simulink model "vegas13_fastnettest_250mhz_r1"  (Simulink 7.4)
settings: Solver=ode45  StartTime=0.0  StopTime=20000  RelTol=1e-3
undefined symbols (not defined in the file or in its folder): ROACH
libraries: xbsIndex_r4 x179, xps_library x20, casper_library_misc x18, dspsigops x16, casper_library_flow_control x4
(part 1 of 3)
settings Model: Creator=dave  LastModifiedBy=sscott
settings OptimizationCC: InitFltsAndDblsToZero=on

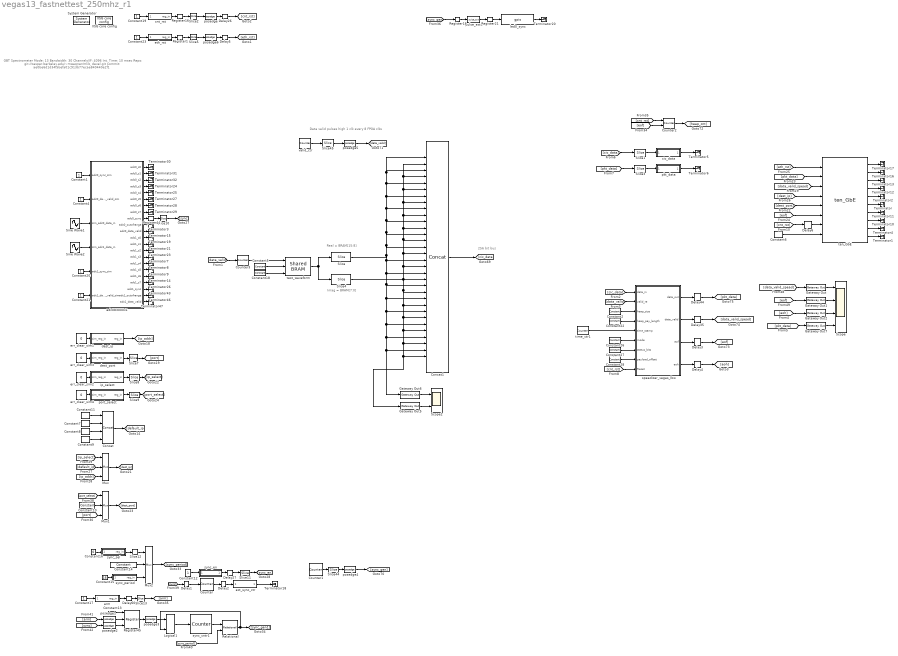
== system vegas13_fastnettest_250mhz_r1 ==
  note: GBT Spectrometer
      | Mode: 13
      | Bandwidth: 30
      | Channels/IF: 4096
      | Int. Time: 10 msec
      | Repo: git://casper.berkeley.edu/~mwagner/mlib_devel.git
      | Commit: ae0be6d1d34f5befa01c913b77ecae840440e2f1
  note: Data valid pulses high 1 clk every 8 FPGA clks
  note: 256 bit bus
  note: Real = BRAM[15:8]
  note: Imag = BRAM[7:0]
  " System Generator" : xbsIndex_r4/ System Generator  Tag=genX  SystemSampleTime=-1  xilinxfamily=virtex5  part=xc5vsx95t  speed=-1  package=ff1136  synthesis_tool=XST  clock_wrapper=Clock Enables  directory=./vegas13_fastnettest_250mhz_r1/sysgen  testbench=off  simulink_period=1  sysclk_period=4  dcm_input_clock_period=100  incr_netlist=off  trim_vbits=Everywhere in SubSystem  dbl_ovrd=According to Block Masks  core_generation=According to Block Masks  run_coregen=off  deprecated_control=off  eval_field=0  block_type=sysgen
      settings: block_version=10.1.3
  Concat : xbsIndex_r4/Concat  num_inputs=4  dbl_ovrd=off  block_type=concat
  Concat1 : xbsIndex_r4/Concat  num_inputs=32  dbl_ovrd=off  block_type=concat
  Constant{1,4,20..21} (4 alike) : Constant  OutDataType=sfix(16)  OutScaling=2^0  SampleTime=1
  Constant10 : xbsIndex_r4/Constant  arith_type=Unsigned  const=10145  n_bits=32  bin_pt=0  explicit_period=on  period=1  equ=P=C  opselect=C  inp2=PCIN>>17  opr=+  inp1=P  carry=CIN  dbl_ovrd=off  block_type=constant
  Constant11 : xbsIndex_r4/Constant  arith_type=Unsigned  const=10  n_bits=8  bin_pt=0  explicit_period=on  period=1  equ=P=C  opselect=C  inp2=PCIN>>17  opr=+  inp1=P  carry=CIN  dbl_ovrd=off  block_type=constant
  Constant12 : Constant  OutDataType=fixdt(1, 16)  OutScaling=2^0
  Constant13 : xbsIndex_r4/Constant  arith_type=Boolean  const=1  n_bits=16  bin_pt=14  explicit_period=on  period=1  equ=P=C  opselect=C  inp2=PCIN>>17  opr=+  inp1=P  carry=CIN  dbl_ovrd=off  block_type=constant
  Constant14 : xbsIndex_r4/Constant  arith_type=Unsigned  const=100663295  n_bits=32  bin_pt=0  explicit_period=on  period=1  equ=P=C  opselect=C  inp2=PCIN>>17  opr=+  inp1=P  carry=CIN  dbl_ovrd=off  block_type=constant
  Constant15 : Constant  Value=16  OutDataType=sfix(16)  OutScaling=2^0
  Constant16 : Constant  Value=0  OutDataType=sfix(16)  OutScaling=2^0
  Constant17 : Constant  OutDataType=sfix(16)  OutScaling=2^0
  Constant{5,18,27..28} (4 alike) : xbsIndex_r4/Constant  arith_type=Unsigned  const=0  n_bits=40  bin_pt=0  explicit_period=on  period=1  equ=P=C  opselect=C  inp2=PCIN>>17  opr=+  inp1=P  carry=CIN  dbl_ovrd=off  block_type=constant
  Constant19 : Constant  OutDataType=sfix(16)  OutScaling=2^0
  Constant2 : xbsIndex_r4/Constant  arith_type=Unsigned  const=8192+4*8  n_bits=40  bin_pt=0  explicit_period=on  period=1  equ=P=C  opselect=C  inp2=PCIN>>17  opr=+  inp1=P  carry=CIN  dbl_ovrd=off  block_type=constant
  Constant22 : xbsIndex_r4/Constant  arith_type=Unsigned  const=8192  n_bits=40  bin_pt=0  explicit_period=on  period=1  equ=P=C  opselect=C  inp2=PCIN>>17  opr=+  inp1=P  carry=CIN  dbl_ovrd=off  block_type=constant
  Constant23 : Constant  OutDataType=sfix(16)  OutScaling=2^0
  Constant26 : xbsIndex_r4/Constant  arith_type=Unsigned  const=13  n_bits=40  bin_pt=0  explicit_period=on  period=1  equ=P=C  opselect=C  inp2=PCIN>>17  opr=+  inp1=P  carry=CIN  dbl_ovrd=off  block_type=constant
  Constant6 : xbsIndex_r4/Constant  arith_type=Boolean  const=0  n_bits=1  bin_pt=0  explicit_period=on  period=1  equ=P=C  opselect=C  inp2=PCIN>>17  opr=+  inp1=P  carry=CIN  dbl_ovrd=off  block_type=constant
  Constant7 : xbsIndex_r4/Constant  arith_type=Unsigned  const=0  n_bits=8  bin_pt=0  explicit_period=on  period=1  equ=P=C  opselect=C  inp2=PCIN>>17  opr=+  inp1=P  carry=CIN  dbl_ovrd=off  block_type=constant
  Constant8 : xbsIndex_r4/Constant  arith_type=Unsigned  const=0  n_bits=8  bin_pt=0  explicit_period=on  period=1  equ=P=C  opselect=C  inp2=PCIN>>17  opr=+  inp1=P  carry=CIN  dbl_ovrd=off  block_type=constant
  Constant9 : xbsIndex_r4/Constant  arith_type=Unsigned  const=145  n_bits=8  bin_pt=0  explicit_period=on  period=1  equ=P=C  opselect=C  inp2=PCIN>>17  opr=+  inp1=P  carry=CIN  dbl_ovrd=off  block_type=constant
  Counter : xbsIndex_r4/Counter  cnt_type=Free Running  cnt_to=Inf  operation=Up  start_count=0  cnt_by_val=1  arith_type=Unsigned  n_bits=8  bin_pt=0  load_pin=off  rst=off  en=on  explicit_period=on  period=1  dbl_ovrd=off  use_behavioral_HDL=off  implementation=Fabric  block_type=counter
      settings: block_version=11.4
  Counter1 : xbsIndex_r4/Counter  cnt_type=Free Running  cnt_to=Inf  operation=Up  start_count=0  cnt_by_val=1  arith_type=Unsigned  n_bits=5  bin_pt=0  load_pin=off  rst=off  en=off  explicit_period=on  period=1  dbl_ovrd=off  use_behavioral_HDL=off  implementation=Fabric  block_type=counter
      settings: block_version=11.4
  Counter2 : xbsIndex_r4/Counter  cnt_type=Free Running  cnt_to=Inf  operation=Up  start_count=0  cnt_by_val=1  arith_type=Unsigned  n_bits=40  bin_pt=0  load_pin=off  rst=on  en=on  explicit_period=on  period=1  dbl_ovrd=off  use_behavioral_HDL=off  implementation=Fabric  block_type=counter
      settings: block_version=11.4
  Counter3 : xbsIndex_r4/Counter  cnt_type=Free Running  cnt_to=Inf  operation=Up  start_count=0  cnt_by_val=1  arith_type=Unsigned  n_bits=4  bin_pt=0  load_pin=off  rst=off  en=on  explicit_period=on  period=1  dbl_ovrd=off  use_behavioral_HDL=off  implementation=Fabric  block_type=counter
      settings: block_version=11.4
  Delay1 : xbsIndex_r4/Delay  en=off  latency=8  dbl_ovrd=off  reg_retiming=off  block_type=delay
      settings: block_version=11.4
  Delay2 : xbsIndex_r4/Delay  en=off  latency=8  dbl_ovrd=off  reg_retiming=off  block_type=delay
      settings: block_version=11.4
  Delay26 : xbsIndex_r4/Delay  en=off  latency=8  dbl_ovrd=off  reg_retiming=on  block_type=delay
  Delay27 : xbsIndex_r4/Delay  en=off  latency=8  dbl_ovrd=off  reg_retiming=off  block_type=delay
      settings: block_version=11.4
  Delay{3..4,6,35,44} (5 alike) : xbsIndex_r4/Delay  en=off  latency=1  dbl_ovrd=off  reg_retiming=on  block_type=delay
  Delay5 : xbsIndex_r4/Delay  en=off  latency=8  dbl_ovrd=off  reg_retiming=on  block_type=delay
  Delay60 : xbsIndex_r4/Delay  en=off  latency=2  dbl_ovrd=off  reg_retiming=on  block_type=delay
  Gateway Out{,1..2,5..7} (6 alike) : xbsIndex_r4/Gateway Out  hdl_port=on  timing_constraint=None  locs_specified=off  LOCs={}  block_type=gatewayout
      settings: infoedit="Gateway out block.  Converts Xilinx fixed point inputs into ouputs of type Simulink integer, double, or fixed point.<br><br>Hardware notes:  In hardware these blocks become top level output ports or are discarded, depending on how they are configured."  block_version=11.4
  Logical1 : xbsIndex_r4/Logical  logical_function=OR  inputs=2  en=off  latency=0  precision=Full  arith_type=Unsigned  n_bits=16  bin_pt=0  align_bp=on  dbl_ovrd=off  block_type=logical
  Mux : xbsIndex_r4/Mux  inputs=2  en=off  latency=0  precision=Full  arith_type=Unsigned  n_bits=16  bin_pt=14  quantization=Truncate  overflow=Wrap  dbl_ovrd=off  block_type=mux
      settings: block_version=11.4
  Mux1 : xbsIndex_r4/Mux  inputs=2  en=off  latency=0  precision=Full  arith_type=Unsigned  n_bits=16  bin_pt=14  quantization=Truncate  overflow=Wrap  dbl_ovrd=off  block_type=mux
      settings: block_version=11.4
  Mux2 : xbsIndex_r4/Mux  inputs=2  en=off  latency=0  precision=Full  arith_type=Unsigned  n_bits=16  bin_pt=14  quantization=Truncate  overflow=Wrap  dbl_ovrd=off  block_type=mux
      settings: block_version=11.4
  Register{1,16,18,21,44} (5 alike) : xbsIndex_r4/Register  init=0  rst=off  en=off  dbl_ovrd=off  block_type=register
      settings: block_version=11.4
  Register45 : xbsIndex_r4/Register  init=0  rst=on  en=on  dbl_ovrd=off  block_type=register
      settings: block_version=11.4
  Relational : xbsIndex_r4/Relational  mode=a>=b  en=off  latency=0  dbl_ovrd=off  block_type=relational
      settings: xl_area=[0, 0, 0, 0, 0, 0, 0]  block_version=9.1.01
  Scope : Scope  NumInputPorts=4
      settings: TimeRange=6000  YMin=0~-1~0~0  YMax=1~1~300000000000000~1e+19  MaxDataPoints=1000000
  Scope2 : Scope  NumInputPorts=2
      settings: YMin=0~-5  YMax=1~5  SaveName=ScopeData3  MaxDataPoints=1000000
  Sine Wave1 : Sin  Amplitude=.9  Bias=0  Frequency=2.*pi/4.  Phase=2*pi*240/200  Samples=10  SampleTime=.0625  Offset=0
  Sine Wave2 : Sin  Amplitude=.9  Bias=0  Frequency=2.*pi/4.  Phase=2*pi*240/200  Samples=10  SampleTime=.0625  Offset=0
  Slice : xbsIndex_r4/Slice  nbits=8  boolean_output=off  mode=Lower Bit Location + Width  bit1=0  base1=MSB of Input  bit0=8  base0=LSB of Input  dbl_ovrd=off  block_type=slice
  Slice1 : xbsIndex_r4/Slice  nbits=32  boolean_output=off  mode=Lower Bit Location + Width  bit1=0  base1=MSB of Input  bit0=0  base0=LSB of Input  dbl_ovrd=off  block_type=slice
  Slice{2,5,8..13} (8 alike) : xbsIndex_r4/Slice  nbits=1  boolean_output=on  mode=Lower Bit Location + Width  bit1=0  base1=MSB of Input  bit0=0  base0=LSB of Input  dbl_ovrd=off  block_type=slice
      Slice10 settings: infoedit="Extracts a given range of bits from each input sample and presents it at the output.  The output type is ordinarily unsigned with binary point at zero, but can be Boolean when the slice is one bit wide.<P><P>Hardware notes: In hardware this block costs nothing."  block_version=10.1.3
      Slice12 settings: block_version=10.1.3
      Slice13 settings: infoedit="Extracts a given range of bits from each input sample and presents it at the output.  The output type is ordinarily unsigned with binary point at zero, but can be Boolean when the slice is one bit wide.<P><P>Hardware notes: In hardware this block costs nothing."  block_version=10.1.3
      Slice2 settings: block_version=10.1.3
      Slice5 settings: block_version=10.1.3
      Slice8 settings: block_version=10.1.3
      Slice9 settings: block_version=10.1.3
  Slice3 : xbsIndex_r4/Slice  nbits=32  boolean_output=off  mode=Lower Bit Location + Width  bit1=0  base1=MSB of Input  bit0=0  base0=LSB of Input  dbl_ovrd=off  block_type=slice
  Slice4 : xbsIndex_r4/Slice  nbits=8  boolean_output=off  mode=Lower Bit Location + Width  bit1=0  base1=LSB of Input  bit0=0  base0=LSB of Input  dbl_ovrd=off  block_type=slice
  Slice44 : xbsIndex_r4/Slice  nbits=1  boolean_output=on  mode=Upper Bit Location + Width  bit1=0  base1=MSB of Input  bit0=0  base0=LSB of Input  dbl_ovrd=off  block_type=slice
  Slice45 : xbsIndex_r4/Slice  nbits=1  boolean_output=on  mode=Upper Bit Location + Width  bit1=0  base1=MSB of Input  bit0=0  base0=LSB of Input  dbl_ovrd=off  block_type=slice
  Slice7 : xbsIndex_r4/Slice  nbits=16  boolean_output=off  mode=Lower Bit Location + Width  bit1=0  base1=MSB of Input  bit0=0  base0=LSB of Input  dbl_ovrd=off  block_type=slice
      settings: infoedit="Extracts a given range of bits from each input sample and presents it at the output.  The output type is ordinarily unsigned with binary point at zero, but can be Boolean when the slice is one bit wide.<P><P>Hardware notes: In hardware this block costs nothing."  block_version=10.1.3
  Terminator{,1..21,23..32,43,46..47} (35 alike) : Terminator
  XSG core config : xps_library/XSG core config  Tag=xps:xsg  SystemSampleTime=-1  hw_sys=ROACH:sx95t  ibob_linux=off  clk_src=adc0_clk  iBOB_clk_src=adc0_clk  BEE2_ctrl_clk_src=sys_clk  BEE2_usr_clk_src=sys_clk  ROACH_clk_src=adc0_clk  CORR_clk_src=sys_clk  gpio_clk_io_group=iBOB:sma  gpio_clk_bit_index=0  clk_rate=250  sample_period=1  synthesis_tool=XST  mpc_type=powerpc440_ext
  adc083000x1 : Subsystem  Tag=xps:adc083000x2  AncestorBlock=xps_library/adc083000x2  mask(adc_083000x2){use_adc0=on, use_adc1=on, demux_adc=off, clock_sync=off, verbose=off, using_ctrl=on, adc_clk_rate=1000, sample_period=1, bit_width=8}
      mask prompts: use_adc0 "Use ZD0K0?"; use_adc1 "Use ZDOK1?"; demux_adc "Demux ADCs by 2?"; clock_sync "Interleave 2 ADC boards?"; verbose "Verbose Block Creation?"; using_ctrl "Add ports for control registers?"; adc_clk_rate "ADC clock rate (MHz)"; sample_period "Sample Period"; bit_width "Output Bit Width"
      mask help:
      | The ADC block converts analog inputs to digital outputs.
      | Every clock cycle, the inputs are sampled and digitized to
      | 8 bit binary point numbers in the range of [-1, 1).
      |
      | Online block-specific documentation: http://casper.berkeley.edu/wiki/Adc083000
      mask init:
      | adc083000_mask;
      mask Help: eval('xlWeb([getenv(''MLIB_ROOT''), ''\doc\html\sys_adc\sys_adc.html''])')
  arm : Subsystem  Tag=xps:sw_reg  mask{io_dir=From Processor, arith_type=Unsigned, bitwidth=32, bin_pt=0, sample_period=1, latency=0}
      link override convert: arith_type=Unsigned  n_bits=32  bin_pt=0
      link override r_spec_2048_r102_cnt_rst_user_data_out: arith_type=Unsigned  n_bits=32  bin_pt=0  period=1
      link override r_spec_2048_r102_nosim_cnt_rst_user_data_out: arith_type=Unsigned  n_bits=32  bin_pt=0  period=1
      link override r_spec_2048_r103_cnt_rst_user_data_out: arith_type=Unsigned  n_bits=32  bin_pt=0  period=1
      link override roach_spec_no10gbe_sync_cnt_rst_user_data_out: arith_type=Unsigned  n_bits=32  bin_pt=0  period=1
      link override roach_spec_rst_cnt_user_data_out: arith_type=Unsigned  n_bits=32  bin_pt=0  period=1
      link override roach_spec_rst_sync_cnt_user_data_out: arith_type=Unsigned  n_bits=32  bin_pt=0  period=1
      mask prompts: io_dir "I/O direction"; arith_type "Data Type"; bitwidth "Data bitwidth"; bin_pt "Data binary point"; sample_period "Sample period"
      mask init:
      | gw_name = clear_name(gcb);
      | config.source = str2func('software_register_init');
      | config.toplevel = gcb;
      | xBlock( config, {io_dir, arith_type, bitwidth, bin_pt, ... 
      |     sample_period, gw_name, latency});
      mask StyleString: popup(From Processor|To Processor),popup(Unsigned|Signed  (2's comp)),edit,edit,edit,edit
  cic_data : Subsystem  Tag=xps:sw_reg  mask{io_dir=To Processor, arith_type=Unsigned, bitwidth=32, bin_pt=0, sample_period=1, latency=0}
      mask prompts: io_dir "I/O direction"; arith_type "Data Type"; bitwidth "Data bitwidth"; bin_pt "Data binary point"; sample_period "Sample period"
      mask init:
      | gw_name = clear_name(gcb);
      | config.source = str2func('software_register_init');
      | config.toplevel = gcb;
      | xBlock( config, {io_dir, arith_type, bitwidth, bin_pt, ... 
      |     sample_period, gw_name, latency});
      mask StyleString: popup(From Processor|To Processor),popup(Unsigned|Signed  (2's comp)),edit,edit,edit,edit
  cnt_rst : Subsystem  Tag=xps:sw_reg  mask{io_dir=From Processor, arith_type=Unsigned, bitwidth=32, bin_pt=0, sample_period=1, latency=0}
      link override convert: arith_type=Unsigned  n_bits=32  bin_pt=0
      link override r_spec_2048_r102_cnt_rst_user_data_out: arith_type=Unsigned  n_bits=32  bin_pt=0  period=1
      link override r_spec_2048_r102_nosim_cnt_rst_user_data_out: arith_type=Unsigned  n_bits=32  bin_pt=0  period=1
      link override r_spec_2048_r103_cnt_rst_user_data_out: arith_type=Unsigned  n_bits=32  bin_pt=0  period=1
      link override roach_spec_no10gbe_sync_cnt_rst_user_data_out: arith_type=Unsigned  n_bits=32  bin_pt=0  period=1
      link override roach_spec_rst_cnt_user_data_out: arith_type=Unsigned  n_bits=32  bin_pt=0  period=1
      link override roach_spec_rst_sync_cnt_user_data_out: arith_type=Unsigned  n_bits=32  bin_pt=0  period=1
      mask prompts: io_dir "I/O direction"; arith_type "Data Type"; bitwidth "Data bitwidth"; bin_pt "Data binary point"; sample_period "Sample period"
      mask init:
      | gw_name = clear_name(gcb);
      | config.source = str2func('software_register_init');
      | config.toplevel = gcb;
      | xBlock( config, {io_dir, arith_type, bitwidth, bin_pt, ... 
      |     sample_period, gw_name, latency});
      mask StyleString: popup(From Processor|To Processor),popup(Unsigned|Signed  (2's comp)),edit,edit,edit,edit
  dest_ip : Subsystem  Tag=xps:sw_reg  mask{io_dir=From Processor, arith_type=Unsigned, bitwidth=32, bin_pt=0, sample_period=1, latency=0}
      link override r_10gbe_demo_dest_ip_user_data_out: arith_type=Unsigned  n_bits=32  bin_pt=0  period=1
      link override r_10gbe_test_dest_ip_user_data_out: arith_type=Unsigned  n_bits=32  bin_pt=0  period=1
      link override r_xaui_test_cnt_rst_user_data_out: arith_type=Unsigned  n_bits=32  bin_pt=0  period=1
      mask prompts: io_dir "I/O direction"; arith_type "Data Type"; bitwidth "Data bitwidth"; bin_pt "Data binary point"; sample_period "Sample period"
      mask init:
      | gw_name = clear_name(gcb);
      | config.source = str2func('software_register_init');
      | config.toplevel = gcb;
      | xBlock( config, {io_dir, arith_type, bitwidth, bin_pt, ... 
      |     sample_period, gw_name, latency});
      mask StyleString: popup(From Processor|To Processor),popup(Unsigned|Signed  (2's comp)),edit,edit,edit,edit
  dest_port : Subsystem  Tag=xps:sw_reg  mask{io_dir=From Processor, arith_type=Unsigned, bitwidth=32, bin_pt=0, sample_period=1, latency=0}
      link override r_10gbe_demo_dest_port_user_data_out: arith_type=Unsigned  n_bits=32  bin_pt=0  period=1
      link override r_10gbe_test_dest_port_user_data_out: arith_type=Unsigned  n_bits=32  bin_pt=0  period=1
      link override r_xaui_test_cnt_rst_user_data_out: arith_type=Unsigned  n_bits=32  bin_pt=0  period=1
      mask prompts: io_dir "I/O direction"; arith_type "Data Type"; bitwidth "Data bitwidth"; bin_pt "Data binary point"; sample_period "Sample period"
      mask init:
      | gw_name = clear_name(gcb);
      | config.source = str2func('software_register_init');
      | config.toplevel = gcb;
      | xBlock( config, {io_dir, arith_type, bitwidth, bin_pt, ... 
      |     sample_period, gw_name, latency});
      mask StyleString: popup(From Processor|To Processor),popup(Unsigned|Signed  (2's comp)),edit,edit,edit,edit
  err_clear_sim{1..4} (4 alike) : Constant  Value=0  OutDataType=sfix(16)  OutScaling=2^0
  eth_rst : Subsystem  Tag=xps:sw_reg  mask{io_dir=From Processor, arith_type=Unsigned, bitwidth=32, bin_pt=0, sample_period=1, latency=0}
      link override convert: arith_type=Unsigned  n_bits=32  bin_pt=0
      link override r_spec_2048_r102_cnt_rst_user_data_out: arith_type=Unsigned  n_bits=32  bin_pt=0  period=1
      link override r_spec_2048_r102_nosim_cnt_rst_user_data_out: arith_type=Unsigned  n_bits=32  bin_pt=0  period=1
      link override r_spec_2048_r103_cnt_rst_user_data_out: arith_type=Unsigned  n_bits=32  bin_pt=0  period=1
      link override roach_spec_no10gbe_sync_cnt_rst_user_data_out: arith_type=Unsigned  n_bits=32  bin_pt=0  period=1
      link override roach_spec_rst_cnt_user_data_out: arith_type=Unsigned  n_bits=32  bin_pt=0  period=1
      link override roach_spec_rst_sync_cnt_user_data_out: arith_type=Unsigned  n_bits=32  bin_pt=0  period=1
      mask prompts: io_dir "I/O direction"; arith_type "Data Type"; bitwidth "Data bitwidth"; bin_pt "Data binary point"; sample_period "Sample period"
      mask init:
      | gw_name = clear_name(gcb);
      | config.source = str2func('software_register_init');
      | config.toplevel = gcb;
      | xBlock( config, {io_dir, arith_type, bitwidth, bin_pt, ... 
      |     sample_period, gw_name, latency});
      mask StyleString: popup(From Processor|To Processor),popup(Unsigned|Signed  (2's comp)),edit,edit,edit,edit
  ext_sync_ctr : Subsystem  Tag=xps:sw_reg  mask{io_dir=To Processor, arith_type=Unsigned, bitwidth=32, bin_pt=0, sample_period=1, latency=0}
      mask prompts: io_dir "I/O direction"; arith_type "Data Type"; bitwidth "Data bitwidth"; bin_pt "Data binary point"; sample_period "Sample period"
      mask init:
      | gw_name = clear_name(gcb);
      | config.source = str2func('software_register_init');
      | config.toplevel = gcb;
      | xBlock( config, {io_dir, arith_type, bitwidth, bin_pt, ... 
      |     sample_period, gw_name, latency});
      mask StyleString: popup(From Processor|To Processor),popup(Unsigned|Signed  (2's comp)),edit,edit,edit,edit
  ip_select : Subsystem  Tag=xps:sw_reg  mask{io_dir=From Processor, arith_type=Unsigned, bitwidth=32, bin_pt=0, sample_period=1, latency=0}
      link override r_10gbe_demo_gbe_core_rst_user_data_out: arith_type=Unsigned  n_bits=32  bin_pt=0  period=1
      link override r_10gbe_test_cnt_rst_user_data_out: arith_type=Unsigned  n_bits=32  bin_pt=0  period=1
      link override r_10gbe_test_gbe_core_rst_user_data_out: arith_type=Unsigned  n_bits=32  bin_pt=0  period=1
      link override r_xaui_test_cnt_rst_user_data_out: arith_type=Unsigned  n_bits=32  bin_pt=0  period=1
      mask prompts: io_dir "I/O direction"; arith_type "Data Type"; bitwidth "Data bitwidth"; bin_pt "Data binary point"; sample_period "Sample period"
      mask init:
      | gw_name = clear_name(gcb);
      | config.source = str2func('software_register_init');
      | config.toplevel = gcb;
      | xBlock( config, {io_dir, arith_type, bitwidth, bin_pt, ... 
      |     sample_period, gw_name, latency});
      mask StyleString: popup(From Processor|To Processor),popup(Unsigned|Signed  (2's comp)),edit,edit,edit,edit
  led0_sync : xps_library/gpio  Tag=xps:gpio  SystemSampleTime=-1  io_group=ROACH:led  io_dir=out  arith_type=Boolean  bitwidth=1  bin_pt=0  bit_index=0  sample_period=1  use_single_ended=off  use_ddr=off  reg_iob=on  reg_clk_phase=0  termination=None
      link override convert: arith_type=Boolean  n_bits=1  bin_pt=0
  pkt_data : Subsystem  Tag=xps:sw_reg  mask{io_dir=To Processor, arith_type=Unsigned, bitwidth=32, bin_pt=0, sample_period=1, latency=0}
      mask prompts: io_dir "I/O direction"; arith_type "Data Type"; bitwidth "Data bitwidth"; bin_pt "Data binary point"; sample_period "Sample period"
      mask init:
      | gw_name = clear_name(gcb);
      | config.source = str2func('software_register_init');
      | config.toplevel = gcb;
      | xBlock( config, {io_dir, arith_type, bitwidth, bin_pt, ... 
      |     sample_period, gw_name, latency});
      mask StyleString: popup(From Processor|To Processor),popup(Unsigned|Signed  (2's comp)),edit,edit,edit,edit
  port_select : Subsystem  Tag=xps:sw_reg  mask{io_dir=From Processor, arith_type=Unsigned, bitwidth=32, bin_pt=0, sample_period=1, latency=0}
      link override r_10gbe_demo_gbe_core_rst_user_data_out: arith_type=Unsigned  n_bits=32  bin_pt=0  period=1
      link override r_10gbe_test_cnt_rst_user_data_out: arith_type=Unsigned  n_bits=32  bin_pt=0  period=1
      link override r_10gbe_test_gbe_core_rst_user_data_out: arith_type=Unsigned  n_bits=32  bin_pt=0  period=1
      link override r_xaui_test_cnt_rst_user_data_out: arith_type=Unsigned  n_bits=32  bin_pt=0  period=1
      mask prompts: io_dir "I/O direction"; arith_type "Data Type"; bitwidth "Data bitwidth"; bin_pt "Data binary point"; sample_period "Sample period"
      mask init:
      | gw_name = clear_name(gcb);
      | config.source = str2func('software_register_init');
      | config.toplevel = gcb;
      | xBlock( config, {io_dir, arith_type, bitwidth, bin_pt, ... 
      |     sample_period, gw_name, latency});
      mask StyleString: popup(From Processor|To Processor),popup(Unsigned|Signed  (2's comp)),edit,edit,edit,edit
  posedge{,1..6} (7 alike) : casper_library_misc/posedge  Tag=Rising Edge Detector  SystemSampleTime=-1
  pulse_ext1 : casper_library_misc/pulse_ext  SystemSampleTime=-1  pulse_len=2^24
  speadizer_vegas_lbw : Subsystem  AncestorBlock=gbt_library/speadizer_vegas_lbw  mask(speadizer_vegas){spead_msw=24, spead_lsw=40, num_items=4, num_payloads=1, pktzr_waste_time=3, data_input_width=256}
      mask prompts: spead_msw "Num bits for SPEAD Item ID"; spead_lsw "Num bits for SPEAD Item value"; num_items "Number of items (+5)"; num_payloads "Number of packets per heap"; pktzr_waste_time "Packetizer waste time"; data_input_width "Data input width"
      mask help:
      | The size of the heap and payload are in Bytes.
      | If there is one packet per heap then payload_offset is 0.
      | All the input must be not longer than 40 bits.
      mask init:
      | speadizer_vegas_init(gcb, 'spead_msw', spead_msw, 'spead_lsw', spead_lsw, 'num_items', num_items, 'num_payloads', num_payloads, 'pktzr_waste_time', pktzr_waste_time, 'data_input_width', data_input_width)
  sync_cntr1 : xbsIndex_r4/Counter  cnt_type=Free Running  cnt_to=1023  operation=Up  start_count=0  cnt_by_val=1  arith_type=Unsigned  n_bits=10  bin_pt=0  load_pin=off  rst=on  en=off  explicit_period=on  period=1  dbl_ovrd=off  use_behavioral_HDL=off  implementation=Fabric  use_rpm=on  block_type=counter
      settings: xl_area=[0, 0, 0, 0, 0, 0, 0]  block_version=9.1.01
  sync_en : Subsystem  Tag=xps:sw_reg  mask{io_dir=From Processor, arith_type=Unsigned, bitwidth=32, bin_pt=0, sample_period=1, latency=0}
      mask prompts: io_dir "I/O direction"; arith_type "Data Type"; bitwidth "Data bitwidth"; bin_pt "Data binary point"; sample_period "Sample period"
      mask init:
      | gw_name = clear_name(gcb);
      | config.source = str2func('software_register_init');
      | config.toplevel = gcb;
      | xBlock( config, {io_dir, arith_type, bitwidth, bin_pt, ... 
      |     sample_period, gw_name, latency});
      mask StyleString: popup(From Processor|To Processor),popup(Unsigned|Signed  (2's comp)),edit,edit,edit,edit
  sync_period : Subsystem  Tag=xps:sw_reg  mask{io_dir=From Processor, arith_type=Unsigned, bitwidth=32, bin_pt=0, sample_period=1, latency=0}
      link override convert: arith_type=Unsigned  n_bits=32  bin_pt=0
      link override r_spec_2048_r102_cnt_rst_user_data_out: arith_type=Unsigned  n_bits=32  bin_pt=0  period=1
      link override r_spec_2048_r102_nosim_cnt_rst_user_data_out: arith_type=Unsigned  n_bits=32  bin_pt=0  period=1
      link override r_spec_2048_r103_cnt_rst_user_data_out: arith_type=Unsigned  n_bits=32  bin_pt=0  period=1
      link override roach_spec_no10gbe_sync_cnt_rst_user_data_out: arith_type=Unsigned  n_bits=32  bin_pt=0  period=1
      link override roach_spec_rst_cnt_user_data_out: arith_type=Unsigned  n_bits=32  bin_pt=0  period=1
      link override roach_spec_rst_sync_cnt_user_data_out: arith_type=Unsigned  n_bits=32  bin_pt=0  period=1
      mask prompts: io_dir "I/O direction"; arith_type "Data Type"; bitwidth "Data bitwidth"; bin_pt "Data binary point"; sample_period "Sample period"
      mask init:
      | gw_name = clear_name(gcb);
      | config.source = str2func('software_register_init');
      | config.toplevel = gcb;
      | xBlock( config, {io_dir, arith_type, bitwidth, bin_pt, ... 
      |     sample_period, gw_name, latency});
      mask StyleString: popup(From Processor|To Processor),popup(Unsigned|Signed  (2's comp)),edit,edit,edit,edit
  sync_sel : Subsystem  Tag=xps:sw_reg  mask{io_dir=From Processor, arith_type=Unsigned, bitwidth=32, bin_pt=0, sample_period=1, latency=0}
      link override convert: arith_type=Unsigned  n_bits=32  bin_pt=0
      link override r_spec_2048_r102_cnt_rst_user_data_out: arith_type=Unsigned  n_bits=32  bin_pt=0  period=1
      link override r_spec_2048_r102_nosim_cnt_rst_user_data_out: arith_type=Unsigned  n_bits=32  bin_pt=0  period=1
      link override r_spec_2048_r103_cnt_rst_user_data_out: arith_type=Unsigned  n_bits=32  bin_pt=0  period=1
      link override roach_spec_no10gbe_sync_cnt_rst_user_data_out: arith_type=Unsigned  n_bits=32  bin_pt=0  period=1
      link override roach_spec_rst_cnt_user_data_out: arith_type=Unsigned  n_bits=32  bin_pt=0  period=1
      link override roach_spec_rst_sync_cnt_user_data_out: arith_type=Unsigned  n_bits=32  bin_pt=0  period=1
      mask prompts: io_dir "I/O direction"; arith_type "Data Type"; bitwidth "Data bitwidth"; bin_pt "Data binary point"; sample_period "Sample period"
      mask init:
      | gw_name = clear_name(gcb);
      | config.source = str2func('software_register_init');
      | config.toplevel = gcb;
      | xBlock( config, {io_dir, arith_type, bitwidth, bin_pt, ... 
      |     sample_period, gw_name, latency});
      mask StyleString: popup(From Processor|To Processor),popup(Unsigned|Signed  (2's comp)),edit,edit,edit,edit
  ten_GbE : xps_library/ten_GbE  Tag=xps:tengbe  SystemSampleTime=-1  port=ROACH:0  mac_lite=off  open_phy=off  show_param=off  pre_emph=3  swing=800  fab_en=off  fab_mac=0  fab_ip=0  fab_udp=0  fab_gate=0
  test_waveform : xps_library/Shared BRAM  Tag=xps:bram  SystemSampleTime=-1  arith_type="Signed  (2's comp)"  addr_width=10  data_width=32  data_bin_pt=0  init_vals=[0:65535]  sample_rate=1
  time_ctr1 : xbsIndex_r4/Counter  cnt_type=Free Running  cnt_to=Inf  operation=Up  start_count=0  cnt_by_val=1  arith_type=Unsigned  n_bits=40  bin_pt=0  load_pin=off  rst=off  en=off  explicit_period=on  period=1  dbl_ovrd=off  use_behavioral_HDL=off  implementation=Fabric  block_type=counter
      settings: block_version=11.4
  valid_ctr : xbsIndex_r4/Counter  cnt_type=Free Running  cnt_to=Inf  operation=Up  start_count=0  cnt_by_val=1  arith_type=Unsigned  n_bits=3  bin_pt=0  load_pin=off  rst=off  en=off  explicit_period=on  period=1  dbl_ovrd=off  use_behavioral_HDL=off  implementation=Fabric  block_type=counter
      settings: block_version=11.4
  wires:
  led0_sync/1 -> Terminator20/1
  pulse_ext1/1 -> Register21/1
  cnt_rst/1(reg_in) -> Register16/1
  Constant19/1 -> cnt_rst/1(sim_reg_in)
  Register16/1 -> Slice2/1
  Slice2/1 -> posedge/1
  [sync_gen] -> Register18/1
  Register21/1 -> led0_sync/1
  Register18/1 -> pulse_ext1/1
  Constant4/1 -> adc083000x1/2(adc0_data_valid_sim)
  Sine Wave1/1 -> adc083000x1/3(sim_adc0_data_in)
  Constant1/1 -> adc083000x1/1(adc0_sync_sim)
  Constant6/1 -> ten_GbE/8
  [eth_rst] -> ten_GbE/1
  err_clear_sim1/1 -> dest_ip/1(sim_reg_in)
  dest_ip/1(reg_in) -> [ip_addr]
  dest_port/1(reg_in) -> Slice7/1
  err_clear_sim3/1 -> dest_port/1(sim_reg_in)
  Slice7/1 -> [port]
  Constant11/1 -> Concat/1
  Constant7/1 -> Concat/2
  Constant8/1 -> Concat/3
  Constant9/1 -> Concat/4
  Concat/1 -> [default_ip]
  [default_ip] -> Mux/2
  Mux/1 -> [dest_ip]
  [ip_addr] -> Mux/3
  err_clear_sim2/1 -> ip_select/1(sim_reg_in)
  ip_select/1(reg_in) -> Slice8/1
  Slice8/1 -> [ip_select]
  [ip_select] -> Mux/1
  Constant10/1 -> Mux1/2
  Mux1/1 -> [dest_port]
  [port] -> Mux1/3
  [port_select] -> Mux1/1
  err_clear_sim4/1 -> port_select/1(sim_reg_in)
  port_select/1(reg_in) -> Slice9/1
  Slice9/1 -> [port_select]
  Slice10/1 -> [sync]
  Register44/1 -> Slice10/1
  Constant12/1 -> sync_en/1(sim_reg_in)
  sync_en/1(reg_in) -> Delay27/1
  Slice11/1 -> [sync_en]
  Delay27/1 -> Slice11/1
  Counter/1 -> Delay2/1
  [sync] -> Delay1/1
  ext_sync_ctr/1(sim_reg_out) -> Terminator18/1
  Delay1/1 -> Counter/1
  Delay2/1 -> ext_sync_ctr/1(reg_out)
  Mux2/1 -> [sync_period]
  Constant15/1 -> sync_period/1(sim_reg_in)
  sync_period/1(reg_in) -> Mux2/3
  Constant14/1 -> Mux2/2
  sync_sel/1(reg_in) -> Slice12/1
  Constant16/1 -> sync_sel/1(sim_reg_in)
  Slice12/1 -> Mux2/1
  Constant13/1 -> Register45/1
  posedge1/1 -> Register45/2
  Register45/1 -> posedge3/1
  posedge3/1 -> Logical1/1
  Logical1/1 -> sync_cntr1/1
  sync_cntr1/1 -> Relational/1
  Relational/1 -> [sync_gen1], Logical1/2
  [arm] -> posedge1/1
  Constant17/1 -> arm/1(sim_reg_in)
  Delay60/1 -> Slice13/1
  arm/1(reg_in) -> Delay60/1
  Slice13/1 -> [arm]
  [sync] -> posedge2/1
  posedge2/1 -> Register45/3
  [sync_period] -> Relational/2
  adc083000x1/9(adc0_sync) -> Register44/1
  adc083000x1/20(adc1_sync) -> Terminator43/1
  adc083000x1/21(adc1_outofrange) -> Terminator46/1
  adc083000x1/22(adc1_data_valid) -> Terminator47/1
  posedge/1 -> Delay26/1
  Sine Wave2/1 -> adc083000x1/4(sim_adc1_data_in)
  Constant20/1 -> adc083000x1/5(adc1_sync_sim)
  Constant21/1 -> adc083000x1/6(adc1_data_valid_sim)
  Delay26/1 -> [cnt_rst]
  adc083000x1/1(adc0_s0) -> Terminator30/1
  adc083000x1/3(adc0_s2) -> Terminator32/1
  adc083000x1/19(adc1_s7) -> Terminator26/1
  adc083000x1/2(adc0_s1) -> Terminator31/1
  adc083000x1/4(adc0_s3) -> Terminator24/1
  adc083000x1/10(adc0_outofrange) -> Terminator3/1
  Concat1/1 -> [cic_data]
  Counter1/1 -> Slice44/1
  Slice44/1 -> posedge4/1
  posedge4/1 -> [sync_gen]
  valid_ctr/1 -> Slice45/1
  Slice45/1 -> posedge5/1
  [eof] -> Counter2/2
  [cnt_rst] -> Counter2/1
  Counter2/1 -> [heap_cnt]
  Gateway Out/1 -> Scope/1
  Gateway Out2/1 -> Scope/3
  Gateway Out1/1 -> Scope/2
  [eoh] -> Gateway Out2/1
  [data_valid_spead] -> Gateway Out/1
  [eof] -> Gateway Out1/1
  posedge5/1 -> [data_valid]
  adc083000x1/18(adc1_s6) -> Terminator14/1
  adc083000x1/17(adc1_s5) -> Terminator9/1
  adc083000x1/16(adc1_s4) -> Terminator8/1
  adc083000x1/11(adc0_data_valid) -> Terminator15/1
  adc083000x1/13(adc1_s1) -> Terminator21/1
  adc083000x1/14(adc1_s2) -> Terminator23/1
  adc083000x1/5(adc0_s4) -> Terminator25/1
  adc083000x1/6(adc0_s5) -> Terminator27/1
  adc083000x1/7(adc0_s6) -> Terminator28/1
  adc083000x1/8(adc0_s7) -> Terminator29/1
  adc083000x1/12(adc1_s0) -> Terminator19/1
  adc083000x1/15(adc1_s3) -> Terminator7/1
  speadizer_vegas_lbw/1(data_out) -> Delay44/1
  speadizer_vegas_lbw/2(data_valid) -> Delay35/1
  [cic_data] -> speadizer_vegas_lbw/1(data_in)
  Constant2/1 -> speadizer_vegas_lbw/3(heap_size)
  Constant22/1 -> speadizer_vegas_lbw/4(heap_pay_length)
  time_ctr1/1 -> speadizer_vegas_lbw/5(time_stamp)
  Constant28/1 -> speadizer_vegas_lbw/8(payload_offset)
  Constant27/1 -> speadizer_vegas_lbw/7(status_bits)
  Constant26/1 -> speadizer_vegas_lbw/6(mode)
  [cnt_rst] -> speadizer_vegas_lbw/9(Reset)
  [data_valid] -> speadizer_vegas_lbw/2(valid_re)
  Gateway Out6/1 -> Scope2/1
  Gateway Out7/1 -> Scope/4
  [pkt_data] -> Gateway Out7/1
  [pkt_data] -> ten_GbE/2
  [dest_ip] -> ten_GbE/4
  [dest_port] -> ten_GbE/5
  ten_GbE/1 -> Terminator17/1
  ten_GbE/2 -> Terminator16/1
  ten_GbE/5 -> Terminator2/1
  ten_GbE/6 -> Terminator/1
  ten_GbE/7 -> Terminator11/1
  ten_GbE/8 -> Terminator10/1
  ten_GbE/9 -> Terminator4/1
  ten_GbE/10 -> Terminator1/1
  cic_data/1(sim_reg_out) -> Terminator5/1
  pkt_data/1(sim_reg_out) -> Terminator6/1
  Slice1/1 -> cic_data/1(reg_out)
  [cic_data] -> Slice1/1
  Slice3/1 -> pkt_data/1(reg_out)
  [pkt_data] -> Slice3/1
  Delay3/1 -> [eof]
  Delay4/1 -> [eoh]
  speadizer_vegas_lbw/3(eof) -> Delay3/1
  speadizer_vegas_lbw/4(eoh) -> Delay4/1
  Delay44/1 -> [pkt_data]
  Delay35/1 -> [data_valid_spead]
  Constant18/1 -> test_waveform/3
  Constant5/1 -> test_waveform/2
  [data_valid] -> Counter3/1
  Counter3/1 -> test_waveform/1
  test_waveform/1 -> Slice/1, Slice4/1
  Slice/1 -> Concat1/1, Concat1/3, Concat1/5, Concat1/7, Concat1/9, Concat1/11, Concat1/13, Concat1/15, Concat1/17, Concat1/19, Concat1/21, Concat1/23, Concat1/25, Concat1/27, Concat1/29, Concat1/31, Gateway Out6/1
  Slice4/1 -> Concat1/20, Concat1/10, Concat1/2, Concat1/4, Concat1/6, Concat1/8, Concat1/12, Concat1/14, Concat1/16, Concat1/18, Concat1/22, Concat1/24, Concat1/26, Concat1/28, Concat1/30, Concat1/32, Gateway Out5/1
  Gateway Out5/1 -> Scope2/2
  eth_rst/1(reg_in) -> Register1/1
  Constant23/1 -> eth_rst/1(sim_reg_in)
  Register1/1 -> Slice5/1
  Slice5/1 -> posedge6/1
  posedge6/1 -> Delay5/1
  Delay5/1 -> [eth_rst]
  [data_valid_spead] -> ten_GbE/3
  [eof] -> ten_GbE/6
  ten_GbE/3 -> Terminator13/1
  ten_GbE/4 -> Terminator12/1
  Delay6/1 -> ten_GbE/7
  [cnt_rst] -> Delay6/1
